simulink model "qless_forgetting_factor_16x16_nofifo"  (R2021a)
settings: Solver=FixedStepDiscrete  StartTime=0.0  StopTime=stoptime*inf  RelTol=1e-3
InitFcn:
  | qless_init_16chan_fi
undefined symbols (not defined in the file): fc, numArrayElements, physconst, srcAngles, Ts
libraries: hdlsllib x137, commfilt2 x4, commrfcorlib x3, commsync2 x3, commrflib2 x2, commrandsrc3 x2, simulink x2, phasedtxrxlib x2, commdigbbndcpm2 x1, embreciprocals x1, commdigbbndpm3 x1
(part 11 of 22)

== system qless_forgetting_factor_16x16_nofifo/MVDR_QLess_HDL/Complex Partial-Systolic Matrix Solve Using Q-less QR Decomposition with Forgetting Factor Manually Tiled n=16/Complex Partial-Systolic Q-less QR with Forgetting Factor/Complex Partial-Systolic Q-less QR with Forgetting Factor Manually tiled/Complex Partial-Systolic Q-less QR Decomposition with Forgetting Factor Section Constant pivot3/Complex Partial-Systolic Q-less QR Row Rotations/Q-less QR Rotate First Element To Real1/Q-less QR Real Row Rotations ==
  x : Inport
  y : Inport  Port=2
  validIn : Inport  Port=3
  restart : Inport  Port=4
  Delay{,1,5..7,10..12,16..18,21} (12 alike) : Delay  DelayLength=1
  Inverse CORDIC Gain : Subsystem  mask(Inverse CORDIC Gain){}
      mask help: fixed:emblib:InverseCORDICGainDescription
      mask Display: disp('1/An')
  Inverse CORDIC Gain1 : Subsystem  mask(Inverse CORDIC Gain){}
      mask help: fixed:emblib:InverseCORDICGainDescription
      mask Display: disp('1/An')
  Q-less QR Real Indexed CORDIC Row Rotation : Subsystem  TreatAsAtomicUnit=on  mask(Real Indexed CORDIC Row Rotation){n=n, pivot=pivot}
      mask prompts: n "fixed:emblib:ColumnsInA"
      mask help: fixed:emblib:RealIdxCORDIC
      mask DialogControl n Prompt: Number of columns in matrix A
  QR 2nd and 3rd Quadrant Compensation : MATLAB Function  TreatAsAtomicUnit=on
  Set Element To Zero : Subsystem  mask(Set Element To Zero){n=n, pivot=pivot}
      mask prompts: n "fixed:emblib:ColumnsInA"
      mask help: fixed:emblib:SetElementToZeroDescription
      mask DialogControl n Prompt: Number of columns in matrix A
  xOut : Outport  VectorParamsAs1DForOutWhenUnconnected=off
  yOut : Outport  Port=2  VectorParamsAs1DForOutWhenUnconnected=off
  validOut : Outport  Port=3  VectorParamsAs1DForOutWhenUnconnected=off
  ready : Outport  Port=4  VectorParamsAs1DForOutWhenUnconnected=off
  wires:
  Delay11/1 -> QR 2nd and 3rd Quadrant Compensation/1(x)
  Delay7/1 -> Set Element To Zero/1(u)
  Delay12/1 -> QR 2nd and 3rd Quadrant Compensation/2(y)
  y/1 -> Delay12/1
  QR 2nd and 3rd Quadrant Compensation/1(xOut) -> Delay/1
  Delay16/1 -> Delay5/1
  Inverse CORDIC Gain1/1(y) -> Delay7/1
  Inverse CORDIC Gain/1(y) -> Delay6/1
  Delay6/1 -> xOut/1
  QR 2nd and 3rd Quadrant Compensation/2(yOut) -> Delay1/1
  x/1 -> Delay11/1
  validIn/1 -> Delay16/1
  Delay17/1 -> Inverse CORDIC Gain/1(u)
  Delay18/1 -> Inverse CORDIC Gain1/1(u)
  Delay21/1 -> Delay10/1
  Set Element To Zero/1(y) -> yOut/1
  Delay10/1 -> validOut/1
  Delay/1 -> Q-less QR Real Indexed CORDIC Row Rotation/1(x)
  Delay1/1 -> Q-less QR Real Indexed CORDIC Row Rotation/2(y)
  Delay5/1 -> Q-less QR Real Indexed CORDIC Row Rotation/3(validIn)
  restart/1 -> Q-less QR Real Indexed CORDIC Row Rotation/4(restart)
  Q-less QR Real Indexed CORDIC Row Rotation/1(xOut) -> Delay17/1
  Q-less QR Real Indexed CORDIC Row Rotation/2(yOut) -> Delay18/1
  Q-less QR Real Indexed CORDIC Row Rotation/3(validOut) -> Delay21/1
  Q-less QR Real Indexed CORDIC Row Rotation/4(ready) -> ready/1

== system qless_forgetting_factor_16x16_nofifo/MVDR_QLess_HDL/Complex Partial-Systolic Matrix Solve Using Q-less QR Decomposition with Forgetting Factor Manually Tiled n=16/Complex Partial-Systolic Q-less QR with Forgetting Factor/Complex Partial-Systolic Q-less QR with Forgetting Factor Manually tiled/Complex Partial-Systolic Q-less QR Decomposition with Forgetting Factor Section Constant pivot3/Complex Partial-Systolic Q-less QR Row Rotations/Q-less QR Rotate First Element To Real1/ValidIn to Ready Logic ==
  readyIn : Inport
  validIn : Inport  Port=2
  AND : Logic  IconShape=distinctive  AllPortsSameDT=off  OutDataTypeStr=boolean
  NOT : Logic  Operator=NOT  IconShape=distinctive  AllPortsSameDT=off  OutDataTypeStr=boolean
  readyOut : Outport  VectorParamsAs1DForOutWhenUnconnected=off
  wires:
  validIn/1 -> NOT/1
  readyIn/1 -> AND/1
  AND/1 -> readyOut/1
  NOT/1 -> AND/2

== system qless_forgetting_factor_16x16_nofifo/MVDR_QLess_HDL/Complex Partial-Systolic Matrix Solve Using Q-less QR Decomposition with Forgetting Factor Manually Tiled n=16/Complex Partial-Systolic Q-less QR with Forgetting Factor/Complex Partial-Systolic Q-less QR with Forgetting Factor Manually tiled/Complex Partial-Systolic Q-less QR Decomposition with Forgetting Factor Section Constant pivot3/Complex Partial-Systolic Q-less QR Row Rotations/Q-less QR Rotate First Element To Real1/ValidIn to Ready Logic1 ==
  readyIn : Inport
  validIn : Inport  Port=2
  AND : Logic  IconShape=distinctive  AllPortsSameDT=off  OutDataTypeStr=boolean
  NOT : Logic  Operator=NOT  IconShape=distinctive  AllPortsSameDT=off  OutDataTypeStr=boolean
  readyOut : Outport  VectorParamsAs1DForOutWhenUnconnected=off
  wires:
  validIn/1 -> NOT/1
  readyIn/1 -> AND/1
  AND/1 -> readyOut/1
  NOT/1 -> AND/2

== system qless_forgetting_factor_16x16_nofifo/MVDR_QLess_HDL/Complex Partial-Systolic Matrix Solve Using Q-less QR Decomposition with Forgetting Factor Manually Tiled n=16/Complex Partial-Systolic Q-less QR with Forgetting Factor/Complex Partial-Systolic Q-less QR with Forgetting Factor Manually tiled/Complex Partial-Systolic Q-less QR Decomposition with Forgetting Factor Section Constant pivot4/Complex Partial-Systolic Q-less QR Row Rotations/Q-less QR Rotate First Element To Real1/Q-less QR Real Row Rotations ==
  x : Inport
  y : Inport  Port=2
  validIn : Inport  Port=3
  restart : Inport  Port=4
  Delay{,1,5..7,10..12,16..18,21} (12 alike) : Delay  DelayLength=1
  Inverse CORDIC Gain : Subsystem  mask(Inverse CORDIC Gain){}
      mask help: fixed:emblib:InverseCORDICGainDescription
      mask Display: disp('1/An')
  Inverse CORDIC Gain1 : Subsystem  mask(Inverse CORDIC Gain){}
      mask help: fixed:emblib:InverseCORDICGainDescription
      mask Display: disp('1/An')
  Q-less QR Real Indexed CORDIC Row Rotation : Subsystem  TreatAsAtomicUnit=on  mask(Real Indexed CORDIC Row Rotation){n=n, pivot=pivot}
      mask prompts: n "fixed:emblib:ColumnsInA"
      mask help: fixed:emblib:RealIdxCORDIC
      mask DialogControl n Prompt: Number of columns in matrix A
  QR 2nd and 3rd Quadrant Compensation : MATLAB Function  TreatAsAtomicUnit=on
  Set Element To Zero : Subsystem  mask(Set Element To Zero){n=n, pivot=pivot}
      mask prompts: n "fixed:emblib:ColumnsInA"
      mask help: fixed:emblib:SetElementToZeroDescription
      mask DialogControl n Prompt: Number of columns in matrix A
  xOut : Outport  VectorParamsAs1DForOutWhenUnconnected=off
  yOut : Outport  Port=2  VectorParamsAs1DForOutWhenUnconnected=off
  validOut : Outport  Port=3  VectorParamsAs1DForOutWhenUnconnected=off
  ready : Outport  Port=4  VectorParamsAs1DForOutWhenUnconnected=off
  wires:
  Delay11/1 -> QR 2nd and 3rd Quadrant Compensation/1(x)
  Delay7/1 -> Set Element To Zero/1(u)
  Delay12/1 -> QR 2nd and 3rd Quadrant Compensation/2(y)
  y/1 -> Delay12/1
  QR 2nd and 3rd Quadrant Compensation/1(xOut) -> Delay/1
  Delay16/1 -> Delay5/1
  Inverse CORDIC Gain1/1(y) -> Delay7/1
  Inverse CORDIC Gain/1(y) -> Delay6/1
  Delay6/1 -> xOut/1
  QR 2nd and 3rd Quadrant Compensation/2(yOut) -> Delay1/1
  x/1 -> Delay11/1
  validIn/1 -> Delay16/1
  Delay17/1 -> Inverse CORDIC Gain/1(u)
  Delay18/1 -> Inverse CORDIC Gain1/1(u)
  Delay21/1 -> Delay10/1
  Set Element To Zero/1(y) -> yOut/1
  Delay10/1 -> validOut/1
  Delay/1 -> Q-less QR Real Indexed CORDIC Row Rotation/1(x)
  Delay1/1 -> Q-less QR Real Indexed CORDIC Row Rotation/2(y)
  Delay5/1 -> Q-less QR Real Indexed CORDIC Row Rotation/3(validIn)
  restart/1 -> Q-less QR Real Indexed CORDIC Row Rotation/4(restart)
  Q-less QR Real Indexed CORDIC Row Rotation/1(xOut) -> Delay17/1
  Q-less QR Real Indexed CORDIC Row Rotation/2(yOut) -> Delay18/1
  Q-less QR Real Indexed CORDIC Row Rotation/3(validOut) -> Delay21/1
  Q-less QR Real Indexed CORDIC Row Rotation/4(ready) -> ready/1

== system qless_forgetting_factor_16x16_nofifo/MVDR_QLess_HDL/Complex Partial-Systolic Matrix Solve Using Q-less QR Decomposition with Forgetting Factor Manually Tiled n=16/Complex Partial-Systolic Q-less QR with Forgetting Factor/Complex Partial-Systolic Q-less QR with Forgetting Factor Manually tiled/Complex Partial-Systolic Q-less QR Decomposition with Forgetting Factor Section Constant pivot4/Complex Partial-Systolic Q-less QR Row Rotations/Q-less QR Rotate First Element To Real1/ValidIn to Ready Logic ==
  readyIn : Inport
  validIn : Inport  Port=2
  AND : Logic  IconShape=distinctive  AllPortsSameDT=off  OutDataTypeStr=boolean
  NOT : Logic  Operator=NOT  IconShape=distinctive  AllPortsSameDT=off  OutDataTypeStr=boolean
  readyOut : Outport  VectorParamsAs1DForOutWhenUnconnected=off
  wires:
  validIn/1 -> NOT/1
  readyIn/1 -> AND/1
  AND/1 -> readyOut/1
  NOT/1 -> AND/2

== system qless_forgetting_factor_16x16_nofifo/MVDR_QLess_HDL/Complex Partial-Systolic Matrix Solve Using Q-less QR Decomposition with Forgetting Factor Manually Tiled n=16/Complex Partial-Systolic Q-less QR with Forgetting Factor/Complex Partial-Systolic Q-less QR with Forgetting Factor Manually tiled/Complex Partial-Systolic Q-less QR Decomposition with Forgetting Factor Section Constant pivot4/Complex Partial-Systolic Q-less QR Row Rotations/Q-less QR Rotate First Element To Real1/ValidIn to Ready Logic1 ==
  readyIn : Inport
  validIn : Inport  Port=2
  AND : Logic  IconShape=distinctive  AllPortsSameDT=off  OutDataTypeStr=boolean
  NOT : Logic  Operator=NOT  IconShape=distinctive  AllPortsSameDT=off  OutDataTypeStr=boolean
  readyOut : Outport  VectorParamsAs1DForOutWhenUnconnected=off
  wires:
  validIn/1 -> NOT/1
  readyIn/1 -> AND/1
  AND/1 -> readyOut/1
  NOT/1 -> AND/2

== system qless_forgetting_factor_16x16_nofifo/MVDR_QLess_HDL/Complex Partial-Systolic Matrix Solve Using Q-less QR Decomposition with Forgetting Factor Manually Tiled n=16/Complex Partial-Systolic Q-less QR with Forgetting Factor/Complex Partial-Systolic Q-less QR with Forgetting Factor Manually tiled/Complex Partial-Systolic Q-less QR Decomposition with Forgetting Factor Section Constant pivot5/Complex Partial-Systolic Q-less QR Row Rotations/Q-less QR Rotate First Element To Real1/Q-less QR Real Row Rotations ==
  x : Inport
  y : Inport  Port=2
  validIn : Inport  Port=3
  restart : Inport  Port=4
  Delay{,1,5..7,10..12,16..18,21} (12 alike) : Delay  DelayLength=1
  Inverse CORDIC Gain : Subsystem  mask(Inverse CORDIC Gain){}
      mask help: fixed:emblib:InverseCORDICGainDescription
      mask Display: disp('1/An')
  Inverse CORDIC Gain1 : Subsystem  mask(Inverse CORDIC Gain){}
      mask help: fixed:emblib:InverseCORDICGainDescription
      mask Display: disp('1/An')
  Q-less QR Real Indexed CORDIC Row Rotation : Subsystem  TreatAsAtomicUnit=on  mask(Real Indexed CORDIC Row Rotation){n=n, pivot=pivot}
      mask prompts: n "fixed:emblib:ColumnsInA"
      mask help: fixed:emblib:RealIdxCORDIC
      mask DialogControl n Prompt: Number of columns in matrix A
  QR 2nd and 3rd Quadrant Compensation : MATLAB Function  TreatAsAtomicUnit=on
  Set Element To Zero : Subsystem  mask(Set Element To Zero){n=n, pivot=pivot}
      mask prompts: n "fixed:emblib:ColumnsInA"
      mask help: fixed:emblib:SetElementToZeroDescription
      mask DialogControl n Prompt: Number of columns in matrix A
  xOut : Outport  VectorParamsAs1DForOutWhenUnconnected=off
  yOut : Outport  Port=2  VectorParamsAs1DForOutWhenUnconnected=off
  validOut : Outport  Port=3  VectorParamsAs1DForOutWhenUnconnected=off
  ready : Outport  Port=4  VectorParamsAs1DForOutWhenUnconnected=off
  wires:
  Delay11/1 -> QR 2nd and 3rd Quadrant Compensation/1(x)
  Delay7/1 -> Set Element To Zero/1(u)
  Delay12/1 -> QR 2nd and 3rd Quadrant Compensation/2(y)
  y/1 -> Delay12/1
  QR 2nd and 3rd Quadrant Compensation/1(xOut) -> Delay/1
  Delay16/1 -> Delay5/1
  Inverse CORDIC Gain1/1(y) -> Delay7/1
  Inverse CORDIC Gain/1(y) -> Delay6/1
  Delay6/1 -> xOut/1
  QR 2nd and 3rd Quadrant Compensation/2(yOut) -> Delay1/1
  x/1 -> Delay11/1
  validIn/1 -> Delay16/1
  Delay17/1 -> Inverse CORDIC Gain/1(u)
  Delay18/1 -> Inverse CORDIC Gain1/1(u)
  Delay21/1 -> Delay10/1
  Set Element To Zero/1(y) -> yOut/1
  Delay10/1 -> validOut/1
  Delay/1 -> Q-less QR Real Indexed CORDIC Row Rotation/1(x)
  Delay1/1 -> Q-less QR Real Indexed CORDIC Row Rotation/2(y)
  Delay5/1 -> Q-less QR Real Indexed CORDIC Row Rotation/3(validIn)
  restart/1 -> Q-less QR Real Indexed CORDIC Row Rotation/4(restart)
  Q-less QR Real Indexed CORDIC Row Rotation/1(xOut) -> Delay17/1
  Q-less QR Real Indexed CORDIC Row Rotation/2(yOut) -> Delay18/1
  Q-less QR Real Indexed CORDIC Row Rotation/3(validOut) -> Delay21/1
  Q-less QR Real Indexed CORDIC Row Rotation/4(ready) -> ready/1

== system qless_forgetting_factor_16x16_nofifo/MVDR_QLess_HDL/Complex Partial-Systolic Matrix Solve Using Q-less QR Decomposition with Forgetting Factor Manually Tiled n=16/Complex Partial-Systolic Q-less QR with Forgetting Factor/Complex Partial-Systolic Q-less QR with Forgetting Factor Manually tiled/Complex Partial-Systolic Q-less QR Decomposition with Forgetting Factor Section Constant pivot5/Complex Partial-Systolic Q-less QR Row Rotations/Q-less QR Rotate First Element To Real1/ValidIn to Ready Logic ==
  readyIn : Inport
  validIn : Inport  Port=2
  AND : Logic  IconShape=distinctive  AllPortsSameDT=off  OutDataTypeStr=boolean
  NOT : Logic  Operator=NOT  IconShape=distinctive  AllPortsSameDT=off  OutDataTypeStr=boolean
  readyOut : Outport  VectorParamsAs1DForOutWhenUnconnected=off
  wires:
  validIn/1 -> NOT/1
  readyIn/1 -> AND/1
  AND/1 -> readyOut/1
  NOT/1 -> AND/2

== system qless_forgetting_factor_16x16_nofifo/MVDR_QLess_HDL/Complex Partial-Systolic Matrix Solve Using Q-less QR Decomposition with Forgetting Factor Manually Tiled n=16/Complex Partial-Systolic Q-less QR with Forgetting Factor/Complex Partial-Systolic Q-less QR with Forgetting Factor Manually tiled/Complex Partial-Systolic Q-less QR Decomposition with Forgetting Factor Section Constant pivot5/Complex Partial-Systolic Q-less QR Row Rotations/Q-less QR Rotate First Element To Real1/ValidIn to Ready Logic1 ==
  readyIn : Inport
  validIn : Inport  Port=2
  AND : Logic  IconShape=distinctive  AllPortsSameDT=off  OutDataTypeStr=boolean
  NOT : Logic  Operator=NOT  IconShape=distinctive  AllPortsSameDT=off  OutDataTypeStr=boolean
  readyOut : Outport  VectorParamsAs1DForOutWhenUnconnected=off
  wires:
  validIn/1 -> NOT/1
  readyIn/1 -> AND/1
  AND/1 -> readyOut/1
  NOT/1 -> AND/2

== system qless_forgetting_factor_16x16_nofifo/MVDR_QLess_HDL/Complex Partial-Systolic Matrix Solve Using Q-less QR Decomposition with Forgetting Factor Manually Tiled n=16/Complex Partial-Systolic Q-less QR with Forgetting Factor/Complex Partial-Systolic Q-less QR with Forgetting Factor Manually tiled/Complex Partial-Systolic Q-less QR Decomposition with Forgetting Factor Section Constant pivot6/Complex Partial-Systolic Q-less QR Row Rotations/Q-less QR Rotate First Element To Real1/Q-less QR Real Row Rotations ==
  x : Inport
  y : Inport  Port=2
  validIn : Inport  Port=3
  restart : Inport  Port=4
  Delay{,1,5..7,10..12,16..18,21} (12 alike) : Delay  DelayLength=1
  Inverse CORDIC Gain : Subsystem  mask(Inverse CORDIC Gain){}
      mask help: fixed:emblib:InverseCORDICGainDescription
      mask Display: disp('1/An')
  Inverse CORDIC Gain1 : Subsystem  mask(Inverse CORDIC Gain){}
      mask help: fixed:emblib:InverseCORDICGainDescription
      mask Display: disp('1/An')
  Q-less QR Real Indexed CORDIC Row Rotation : Subsystem  TreatAsAtomicUnit=on  mask(Real Indexed CORDIC Row Rotation){n=n, pivot=pivot}
      mask prompts: n "fixed:emblib:ColumnsInA"
      mask help: fixed:emblib:RealIdxCORDIC
      mask DialogControl n Prompt: Number of columns in matrix A
  QR 2nd and 3rd Quadrant Compensation : MATLAB Function  TreatAsAtomicUnit=on
  Set Element To Zero : Subsystem  mask(Set Element To Zero){n=n, pivot=pivot}
      mask prompts: n "fixed:emblib:ColumnsInA"
      mask help: fixed:emblib:SetElementToZeroDescription
      mask DialogControl n Prompt: Number of columns in matrix A
  xOut : Outport  VectorParamsAs1DForOutWhenUnconnected=off
  yOut : Outport  Port=2  VectorParamsAs1DForOutWhenUnconnected=off
  validOut : Outport  Port=3  VectorParamsAs1DForOutWhenUnconnected=off
  ready : Outport  Port=4  VectorParamsAs1DForOutWhenUnconnected=off
  wires:
  Delay11/1 -> QR 2nd and 3rd Quadrant Compensation/1(x)
  Delay7/1 -> Set Element To Zero/1(u)
  Delay12/1 -> QR 2nd and 3rd Quadrant Compensation/2(y)
  y/1 -> Delay12/1
  QR 2nd and 3rd Quadrant Compensation/1(xOut) -> Delay/1
  Delay16/1 -> Delay5/1
  Inverse CORDIC Gain1/1(y) -> Delay7/1
  Inverse CORDIC Gain/1(y) -> Delay6/1
  Delay6/1 -> xOut/1
  QR 2nd and 3rd Quadrant Compensation/2(yOut) -> Delay1/1
  x/1 -> Delay11/1
  validIn/1 -> Delay16/1
  Delay17/1 -> Inverse CORDIC Gain/1(u)
  Delay18/1 -> Inverse CORDIC Gain1/1(u)
  Delay21/1 -> Delay10/1
  Set Element To Zero/1(y) -> yOut/1
  Delay10/1 -> validOut/1
  Delay/1 -> Q-less QR Real Indexed CORDIC Row Rotation/1(x)
  Delay1/1 -> Q-less QR Real Indexed CORDIC Row Rotation/2(y)
  Delay5/1 -> Q-less QR Real Indexed CORDIC Row Rotation/3(validIn)
  restart/1 -> Q-less QR Real Indexed CORDIC Row Rotation/4(restart)
  Q-less QR Real Indexed CORDIC Row Rotation/1(xOut) -> Delay17/1
  Q-less QR Real Indexed CORDIC Row Rotation/2(yOut) -> Delay18/1
  Q-less QR Real Indexed CORDIC Row Rotation/3(validOut) -> Delay21/1
  Q-less QR Real Indexed CORDIC Row Rotation/4(ready) -> ready/1

== system qless_forgetting_factor_16x16_nofifo/MVDR_QLess_HDL/Complex Partial-Systolic Matrix Solve Using Q-less QR Decomposition with Forgetting Factor Manually Tiled n=16/Complex Partial-Systolic Q-less QR with Forgetting Factor/Complex Partial-Systolic Q-less QR with Forgetting Factor Manually tiled/Complex Partial-Systolic Q-less QR Decomposition with Forgetting Factor Section Constant pivot6/Complex Partial-Systolic Q-less QR Row Rotations/Q-less QR Rotate First Element To Real1/ValidIn to Ready Logic ==
  readyIn : Inport
  validIn : Inport  Port=2
  AND : Logic  IconShape=distinctive  AllPortsSameDT=off  OutDataTypeStr=boolean
  NOT : Logic  Operator=NOT  IconShape=distinctive  AllPortsSameDT=off  OutDataTypeStr=boolean
  readyOut : Outport  VectorParamsAs1DForOutWhenUnconnected=off
  wires:
  validIn/1 -> NOT/1
  readyIn/1 -> AND/1
  AND/1 -> readyOut/1
  NOT/1 -> AND/2

== system qless_forgetting_factor_16x16_nofifo/MVDR_QLess_HDL/Complex Partial-Systolic Matrix Solve Using Q-less QR Decomposition with Forgetting Factor Manually Tiled n=16/Complex Partial-Systolic Q-less QR with Forgetting Factor/Complex Partial-Systolic Q-less QR with Forgetting Factor Manually tiled/Complex Partial-Systolic Q-less QR Decomposition with Forgetting Factor Section Constant pivot6/Complex Partial-Systolic Q-less QR Row Rotations/Q-less QR Rotate First Element To Real1/ValidIn to Ready Logic1 ==
  readyIn : Inport
  validIn : Inport  Port=2
  AND : Logic  IconShape=distinctive  AllPortsSameDT=off  OutDataTypeStr=boolean
  NOT : Logic  Operator=NOT  IconShape=distinctive  AllPortsSameDT=off  OutDataTypeStr=boolean
  readyOut : Outport  VectorParamsAs1DForOutWhenUnconnected=off
  wires:
  validIn/1 -> NOT/1
  readyIn/1 -> AND/1
  AND/1 -> readyOut/1
  NOT/1 -> AND/2

== system qless_forgetting_factor_16x16_nofifo/MVDR_QLess_HDL/Complex Partial-Systolic Matrix Solve Using Q-less QR Decomposition with Forgetting Factor Manually Tiled n=16/Complex Partial-Systolic Q-less QR with Forgetting Factor/Complex Partial-Systolic Q-less QR with Forgetting Factor Manually tiled/Complex Partial-Systolic Q-less QR Decomposition with Forgetting Factor Section Constant pivot7/Complex Partial-Systolic Q-less QR Row Rotations/Q-less QR Rotate First Element To Real1/Q-less QR Real Row Rotations ==
  x : Inport
  y : Inport  Port=2
  validIn : Inport  Port=3
  restart : Inport  Port=4
  Delay{,1,5..7,10..12,16..18,21} (12 alike) : Delay  DelayLength=1
  Inverse CORDIC Gain : Subsystem  mask(Inverse CORDIC Gain){}
      mask help: fixed:emblib:InverseCORDICGainDescription
      mask Display: disp('1/An')
  Inverse CORDIC Gain1 : Subsystem  mask(Inverse CORDIC Gain){}
      mask help: fixed:emblib:InverseCORDICGainDescription
      mask Display: disp('1/An')
  Q-less QR Real Indexed CORDIC Row Rotation : Subsystem  TreatAsAtomicUnit=on  mask(Real Indexed CORDIC Row Rotation){n=n, pivot=pivot}
      mask prompts: n "fixed:emblib:ColumnsInA"
      mask help: fixed:emblib:RealIdxCORDIC
      mask DialogControl n Prompt: Number of columns in matrix A
  QR 2nd and 3rd Quadrant Compensation : MATLAB Function  TreatAsAtomicUnit=on
  Set Element To Zero : Subsystem  mask(Set Element To Zero){n=n, pivot=pivot}
      mask prompts: n "fixed:emblib:ColumnsInA"
      mask help: fixed:emblib:SetElementToZeroDescription
      mask DialogControl n Prompt: Number of columns in matrix A
  xOut : Outport  VectorParamsAs1DForOutWhenUnconnected=off
  yOut : Outport  Port=2  VectorParamsAs1DForOutWhenUnconnected=off
  validOut : Outport  Port=3  VectorParamsAs1DForOutWhenUnconnected=off
  ready : Outport  Port=4  VectorParamsAs1DForOutWhenUnconnected=off
  wires:
  Delay11/1 -> QR 2nd and 3rd Quadrant Compensation/1(x)
  Delay7/1 -> Set Element To Zero/1(u)
  Delay12/1 -> QR 2nd and 3rd Quadrant Compensation/2(y)
  y/1 -> Delay12/1
  QR 2nd and 3rd Quadrant Compensation/1(xOut) -> Delay/1
  Delay16/1 -> Delay5/1
  Inverse CORDIC Gain1/1(y) -> Delay7/1
  Inverse CORDIC Gain/1(y) -> Delay6/1
  Delay6/1 -> xOut/1
  QR 2nd and 3rd Quadrant Compensation/2(yOut) -> Delay1/1
  x/1 -> Delay11/1
  validIn/1 -> Delay16/1
  Delay17/1 -> Inverse CORDIC Gain/1(u)
  Delay18/1 -> Inverse CORDIC Gain1/1(u)
  Delay21/1 -> Delay10/1
  Set Element To Zero/1(y) -> yOut/1
  Delay10/1 -> validOut/1
  Delay/1 -> Q-less QR Real Indexed CORDIC Row Rotation/1(x)
  Delay1/1 -> Q-less QR Real Indexed CORDIC Row Rotation/2(y)
  Delay5/1 -> Q-less QR Real Indexed CORDIC Row Rotation/3(validIn)
  restart/1 -> Q-less QR Real Indexed CORDIC Row Rotation/4(restart)
  Q-less QR Real Indexed CORDIC Row Rotation/1(xOut) -> Delay17/1
  Q-less QR Real Indexed CORDIC Row Rotation/2(yOut) -> Delay18/1
  Q-less QR Real Indexed CORDIC Row Rotation/3(validOut) -> Delay21/1
  Q-less QR Real Indexed CORDIC Row Rotation/4(ready) -> ready/1

== system qless_forgetting_factor_16x16_nofifo/MVDR_QLess_HDL/Complex Partial-Systolic Matrix Solve Using Q-less QR Decomposition with Forgetting Factor Manually Tiled n=16/Complex Partial-Systolic Q-less QR with Forgetting Factor/Complex Partial-Systolic Q-less QR with Forgetting Factor Manually tiled/Complex Partial-Systolic Q-less QR Decomposition with Forgetting Factor Section Constant pivot7/Complex Partial-Systolic Q-less QR Row Rotations/Q-less QR Rotate First Element To Real1/ValidIn to Ready Logic ==
  readyIn : Inport
  validIn : Inport  Port=2
  AND : Logic  IconShape=distinctive  AllPortsSameDT=off  OutDataTypeStr=boolean
  NOT : Logic  Operator=NOT  IconShape=distinctive  AllPortsSameDT=off  OutDataTypeStr=boolean
  readyOut : Outport  VectorParamsAs1DForOutWhenUnconnected=off
  wires:
  validIn/1 -> NOT/1
  readyIn/1 -> AND/1
  AND/1 -> readyOut/1
  NOT/1 -> AND/2

== system qless_forgetting_factor_16x16_nofifo/MVDR_QLess_HDL/Complex Partial-Systolic Matrix Solve Using Q-less QR Decomposition with Forgetting Factor Manually Tiled n=16/Complex Partial-Systolic Q-less QR with Forgetting Factor/Complex Partial-Systolic Q-less QR with Forgetting Factor Manually tiled/Complex Partial-Systolic Q-less QR Decomposition with Forgetting Factor Section Constant pivot7/Complex Partial-Systolic Q-less QR Row Rotations/Q-less QR Rotate First Element To Real1/ValidIn to Ready Logic1 ==
  readyIn : Inport
  validIn : Inport  Port=2
  AND : Logic  IconShape=distinctive  AllPortsSameDT=off  OutDataTypeStr=boolean
  NOT : Logic  Operator=NOT  IconShape=distinctive  AllPortsSameDT=off  OutDataTypeStr=boolean
  readyOut : Outport  VectorParamsAs1DForOutWhenUnconnected=off
  wires:
  validIn/1 -> NOT/1
  readyIn/1 -> AND/1
  AND/1 -> readyOut/1
  NOT/1 -> AND/2

== system qless_forgetting_factor_16x16_nofifo/MVDR_QLess_HDL/Complex Partial-Systolic Matrix Solve Using Q-less QR Decomposition with Forgetting Factor Manually Tiled n=16/Complex Partial-Systolic Q-less QR with Forgetting Factor/Complex Partial-Systolic Q-less QR with Forgetting Factor Manually tiled/Complex Partial-Systolic Q-less QR Decomposition with Forgetting Factor Section Constant pivot8/Complex Partial-Systolic Q-less QR Row Rotations/Q-less QR Rotate First Element To Real1/Q-less QR Real Row Rotations ==
  x : Inport
  y : Inport  Port=2
  validIn : Inport  Port=3
  restart : Inport  Port=4
  Delay{,1,5..7,10..12,16..18,21} (12 alike) : Delay  DelayLength=1
  Inverse CORDIC Gain : Subsystem  mask(Inverse CORDIC Gain){}
      mask help: fixed:emblib:InverseCORDICGainDescription
      mask Display: disp('1/An')
  Inverse CORDIC Gain1 : Subsystem  mask(Inverse CORDIC Gain){}
      mask help: fixed:emblib:InverseCORDICGainDescription
      mask Display: disp('1/An')
  Q-less QR Real Indexed CORDIC Row Rotation : Subsystem  TreatAsAtomicUnit=on  mask(Real Indexed CORDIC Row Rotation){n=n, pivot=pivot}
      mask prompts: n "fixed:emblib:ColumnsInA"
      mask help: fixed:emblib:RealIdxCORDIC
      mask DialogControl n Prompt: Number of columns in matrix A
  QR 2nd and 3rd Quadrant Compensation : MATLAB Function  TreatAsAtomicUnit=on
  Set Element To Zero : Subsystem  mask(Set Element To Zero){n=n, pivot=pivot}
      mask prompts: n "fixed:emblib:ColumnsInA"
      mask help: fixed:emblib:SetElementToZeroDescription
      mask DialogControl n Prompt: Number of columns in matrix A
  xOut : Outport  VectorParamsAs1DForOutWhenUnconnected=off
  yOut : Outport  Port=2  VectorParamsAs1DForOutWhenUnconnected=off
  validOut : Outport  Port=3  VectorParamsAs1DForOutWhenUnconnected=off
  ready : Outport  Port=4  VectorParamsAs1DForOutWhenUnconnected=off
  wires:
  Delay11/1 -> QR 2nd and 3rd Quadrant Compensation/1(x)
  Delay7/1 -> Set Element To Zero/1(u)
  Delay12/1 -> QR 2nd and 3rd Quadrant Compensation/2(y)
  y/1 -> Delay12/1
  QR 2nd and 3rd Quadrant Compensation/1(xOut) -> Delay/1
  Delay16/1 -> Delay5/1
  Inverse CORDIC Gain1/1(y) -> Delay7/1
  Inverse CORDIC Gain/1(y) -> Delay6/1
  Delay6/1 -> xOut/1
  QR 2nd and 3rd Quadrant Compensation/2(yOut) -> Delay1/1
  x/1 -> Delay11/1
  validIn/1 -> Delay16/1
  Delay17/1 -> Inverse CORDIC Gain/1(u)
  Delay18/1 -> Inverse CORDIC Gain1/1(u)
  Delay21/1 -> Delay10/1
  Set Element To Zero/1(y) -> yOut/1
  Delay10/1 -> validOut/1
  Delay/1 -> Q-less QR Real Indexed CORDIC Row Rotation/1(x)
  Delay1/1 -> Q-less QR Real Indexed CORDIC Row Rotation/2(y)
  Delay5/1 -> Q-less QR Real Indexed CORDIC Row Rotation/3(validIn)
  restart/1 -> Q-less QR Real Indexed CORDIC Row Rotation/4(restart)
  Q-less QR Real Indexed CORDIC Row Rotation/1(xOut) -> Delay17/1
  Q-less QR Real Indexed CORDIC Row Rotation/2(yOut) -> Delay18/1
  Q-less QR Real Indexed CORDIC Row Rotation/3(validOut) -> Delay21/1
  Q-less QR Real Indexed CORDIC Row Rotation/4(ready) -> ready/1

== system qless_forgetting_factor_16x16_nofifo/MVDR_QLess_HDL/Complex Partial-Systolic Matrix Solve Using Q-less QR Decomposition with Forgetting Factor Manually Tiled n=16/Complex Partial-Systolic Q-less QR with Forgetting Factor/Complex Partial-Systolic Q-less QR with Forgetting Factor Manually tiled/Complex Partial-Systolic Q-less QR Decomposition with Forgetting Factor Section Constant pivot8/Complex Partial-Systolic Q-less QR Row Rotations/Q-less QR Rotate First Element To Real1/ValidIn to Ready Logic ==
  readyIn : Inport
  validIn : Inport  Port=2
  AND : Logic  IconShape=distinctive  AllPortsSameDT=off  OutDataTypeStr=boolean
  NOT : Logic  Operator=NOT  IconShape=distinctive  AllPortsSameDT=off  OutDataTypeStr=boolean
  readyOut : Outport  VectorParamsAs1DForOutWhenUnconnected=off
  wires:
  validIn/1 -> NOT/1
  readyIn/1 -> AND/1
  AND/1 -> readyOut/1
  NOT/1 -> AND/2

== system qless_forgetting_factor_16x16_nofifo/MVDR_QLess_HDL/Complex Partial-Systolic Matrix Solve Using Q-less QR Decomposition with Forgetting Factor Manually Tiled n=16/Complex Partial-Systolic Q-less QR with Forgetting Factor/Complex Partial-Systolic Q-less QR with Forgetting Factor Manually tiled/Complex Partial-Systolic Q-less QR Decomposition with Forgetting Factor Section Constant pivot8/Complex Partial-Systolic Q-less QR Row Rotations/Q-less QR Rotate First Element To Real1/ValidIn to Ready Logic1 ==
  readyIn : Inport
  validIn : Inport  Port=2
  AND : Logic  IconShape=distinctive  AllPortsSameDT=off  OutDataTypeStr=boolean
  NOT : Logic  Operator=NOT  IconShape=distinctive  AllPortsSameDT=off  OutDataTypeStr=boolean
  readyOut : Outport  VectorParamsAs1DForOutWhenUnconnected=off
  wires:
  validIn/1 -> NOT/1
  readyIn/1 -> AND/1
  AND/1 -> readyOut/1
  NOT/1 -> AND/2

== system qless_forgetting_factor_16x16_nofifo/MVDR_QLess_HDL/Complex Partial-Systolic Matrix Solve Using Q-less QR Decomposition with Forgetting Factor Manually Tiled n=16/Complex Partial-Systolic Q-less QR with Forgetting Factor/Complex Partial-Systolic Q-less QR with Forgetting Factor Manually tiled/Complex Partial-Systolic Q-less QR Decomposition with Forgetting Factor Section Constant pivot9/Complex Partial-Systolic Q-less QR Row Rotations/Q-less QR Rotate First Element To Real1/Q-less QR Real Row Rotations ==
  x : Inport
  y : Inport  Port=2
  validIn : Inport  Port=3
  restart : Inport  Port=4
  Delay{,1,5..7,10..12,16..18,21} (12 alike) : Delay  DelayLength=1
  Inverse CORDIC Gain : Subsystem  mask(Inverse CORDIC Gain){}
      mask help: fixed:emblib:InverseCORDICGainDescription
      mask Display: disp('1/An')
  Inverse CORDIC Gain1 : Subsystem  mask(Inverse CORDIC Gain){}
      mask help: fixed:emblib:InverseCORDICGainDescription
      mask Display: disp('1/An')
  Q-less QR Real Indexed CORDIC Row Rotation : Subsystem  TreatAsAtomicUnit=on  mask(Real Indexed CORDIC Row Rotation){n=n, pivot=pivot}
      mask prompts: n "fixed:emblib:ColumnsInA"
      mask help: fixed:emblib:RealIdxCORDIC
      mask DialogControl n Prompt: Number of columns in matrix A
  QR 2nd and 3rd Quadrant Compensation : MATLAB Function  TreatAsAtomicUnit=on
  Set Element To Zero : Subsystem  mask(Set Element To Zero){n=n, pivot=pivot}
      mask prompts: n "fixed:emblib:ColumnsInA"
      mask help: fixed:emblib:SetElementToZeroDescription
      mask DialogControl n Prompt: Number of columns in matrix A
  xOut : Outport  VectorParamsAs1DForOutWhenUnconnected=off
  yOut : Outport  Port=2  VectorParamsAs1DForOutWhenUnconnected=off
  validOut : Outport  Port=3  VectorParamsAs1DForOutWhenUnconnected=off
  ready : Outport  Port=4  VectorParamsAs1DForOutWhenUnconnected=off
  wires:
  Delay11/1 -> QR 2nd and 3rd Quadrant Compensation/1(x)
  Delay7/1 -> Set Element To Zero/1(u)
  Delay12/1 -> QR 2nd and 3rd Quadrant Compensation/2(y)
  y/1 -> Delay12/1
  QR 2nd and 3rd Quadrant Compensation/1(xOut) -> Delay/1
  Delay16/1 -> Delay5/1
  Inverse CORDIC Gain1/1(y) -> Delay7/1
  Inverse CORDIC Gain/1(y) -> Delay6/1
  Delay6/1 -> xOut/1
  QR 2nd and 3rd Quadrant Compensation/2(yOut) -> Delay1/1
  x/1 -> Delay11/1
  validIn/1 -> Delay16/1
  Delay17/1 -> Inverse CORDIC Gain/1(u)
  Delay18/1 -> Inverse CORDIC Gain1/1(u)
  Delay21/1 -> Delay10/1
  Set Element To Zero/1(y) -> yOut/1
  Delay10/1 -> validOut/1
  Delay/1 -> Q-less QR Real Indexed CORDIC Row Rotation/1(x)
  Delay1/1 -> Q-less QR Real Indexed CORDIC Row Rotation/2(y)
  Delay5/1 -> Q-less QR Real Indexed CORDIC Row Rotation/3(validIn)
  restart/1 -> Q-less QR Real Indexed CORDIC Row Rotation/4(restart)
  Q-less QR Real Indexed CORDIC Row Rotation/1(xOut) -> Delay17/1
  Q-less QR Real Indexed CORDIC Row Rotation/2(yOut) -> Delay18/1
  Q-less QR Real Indexed CORDIC Row Rotation/3(validOut) -> Delay21/1
  Q-less QR Real Indexed CORDIC Row Rotation/4(ready) -> ready/1

== system qless_forgetting_factor_16x16_nofifo/MVDR_QLess_HDL/Complex Partial-Systolic Matrix Solve Using Q-less QR Decomposition with Forgetting Factor Manually Tiled n=16/Complex Partial-Systolic Q-less QR with Forgetting Factor/Complex Partial-Systolic Q-less QR with Forgetting Factor Manually tiled/Complex Partial-Systolic Q-less QR Decomposition with Forgetting Factor Section Constant pivot9/Complex Partial-Systolic Q-less QR Row Rotations/Q-less QR Rotate First Element To Real1/ValidIn to Ready Logic ==
  readyIn : Inport
  validIn : Inport  Port=2
  AND : Logic  IconShape=distinctive  AllPortsSameDT=off  OutDataTypeStr=boolean
  NOT : Logic  Operator=NOT  IconShape=distinctive  AllPortsSameDT=off  OutDataTypeStr=boolean
  readyOut : Outport  VectorParamsAs1DForOutWhenUnconnected=off
  wires:
  validIn/1 -> NOT/1
  readyIn/1 -> AND/1
  AND/1 -> readyOut/1
  NOT/1 -> AND/2

== system qless_forgetting_factor_16x16_nofifo/MVDR_QLess_HDL/Complex Partial-Systolic Matrix Solve Using Q-less QR Decomposition with Forgetting Factor Manually Tiled n=16/Complex Partial-Systolic Q-less QR with Forgetting Factor/Complex Partial-Systolic Q-less QR with Forgetting Factor Manually tiled/Complex Partial-Systolic Q-less QR Decomposition with Forgetting Factor Section Constant pivot9/Complex Partial-Systolic Q-less QR Row Rotations/Q-less QR Rotate First Element To Real1/ValidIn to Ready Logic1 ==
  readyIn : Inport
  validIn : Inport  Port=2
  AND : Logic  IconShape=distinctive  AllPortsSameDT=off  OutDataTypeStr=boolean
  NOT : Logic  Operator=NOT  IconShape=distinctive  AllPortsSameDT=off  OutDataTypeStr=boolean
  readyOut : Outport  VectorParamsAs1DForOutWhenUnconnected=off
  wires:
  validIn/1 -> NOT/1
  readyIn/1 -> AND/1
  AND/1 -> readyOut/1
  NOT/1 -> AND/2

== system qless_forgetting_factor_16x16_nofifo/MVDR_QLess_HDL/Complex Partial-Systolic Matrix Solve Using Q-less QR Decomposition with Forgetting Factor Manually Tiled n=16/Complex Partial-Systolic Q-less QR with Forgetting Factor/Complex Partial-Systolic Q-less QR with Forgetting Factor Manually tiled/Complex Partial-Systolic Q-less QR Decomposition with Forgetting Factor Section Constant pivot1/Complex Partial-Systolic Q-less QR Row Rotations/Q-less QR Rotate First Element To Real1/Q-less QR Real Row Rotations/Inverse CORDIC Gain ==
  u : Inport
  MATLAB Function : MATLAB Function  TreatAsAtomicUnit=on
  y : Outport  VectorParamsAs1DForOutWhenUnconnected=off
  wires:
  MATLAB Function/1(y) -> y/1
  u/1 -> MATLAB Function/1(u)

== system qless_forgetting_factor_16x16_nofifo/MVDR_QLess_HDL/Complex Partial-Systolic Matrix Solve Using Q-less QR Decomposition with Forgetting Factor Manually Tiled n=16/Complex Partial-Systolic Q-less QR with Forgetting Factor/Complex Partial-Systolic Q-less QR with Forgetting Factor Manually tiled/Complex Partial-Systolic Q-less QR Decomposition with Forgetting Factor Section Constant pivot1/Complex Partial-Systolic Q-less QR Row Rotations/Q-less QR Rotate First Element To Real1/Q-less QR Real Row Rotations/Inverse CORDIC Gain1 ==
  u : Inport
  MATLAB Function : MATLAB Function  TreatAsAtomicUnit=on
  y : Outport  VectorParamsAs1DForOutWhenUnconnected=off
  wires:
  MATLAB Function/1(y) -> y/1
  u/1 -> MATLAB Function/1(u)

== system qless_forgetting_factor_16x16_nofifo/MVDR_QLess_HDL/Complex Partial-Systolic Matrix Solve Using Q-less QR Decomposition with Forgetting Factor Manually Tiled n=16/Complex Partial-Systolic Q-less QR with Forgetting Factor/Complex Partial-Systolic Q-less QR with Forgetting Factor Manually tiled/Complex Partial-Systolic Q-less QR Decomposition with Forgetting Factor Section Constant pivot1/Complex Partial-Systolic Q-less QR Row Rotations/Q-less QR Rotate First Element To Real1/Q-less QR Real Row Rotations/Q-less QR Real Indexed CORDIC Row Rotation ==
  x : Inport
  y : Inport  Port=2
  validIn : Inport  Port=3
  restart : Inport  Port=4
  CORDIC QR Kernel : MATLAB Function  TreatAsAtomicUnit=on
  Delay{1..3,6} (4 alike) : Delay  DelayLength=1
  State Control : StateControl  StateControl=Synchronous
  Unit Delay Enabled Synchronous1 : hdlsllib/Discrete/Unit Delay Enabled Synchronous  InitialCondition=0.0  SampleTime=-1
      settings: SourceProductBaseCode=SL
  Unit Delay Enabled Synchronous4 : hdlsllib/Discrete/Unit Delay Enabled Synchronous  InitialCondition=0.0  SampleTime=-1
      settings: SourceProductBaseCode=SL
  xOut : Outport  VectorParamsAs1DForOutWhenUnconnected=off
  yOut : Outport  Port=2  VectorParamsAs1DForOutWhenUnconnected=off
  validOut : Outport  Port=3  VectorParamsAs1DForOutWhenUnconnected=off
  ready : Outport  Port=4  VectorParamsAs1DForOutWhenUnconnected=off
  wires:
  Delay6/1 -> CORDIC QR Kernel/3(validIn)
  Delay2/1 -> CORDIC QR Kernel/2(yIn)
  Delay1/1 -> CORDIC QR Kernel/1(xIn)
  CORDIC QR Kernel/4(ready) -> ready/1
  CORDIC QR Kernel/3(validOut) -> Unit Delay Enabled Synchronous1/2, Unit Delay Enabled Synchronous4/2, Delay3/1
  restart/1 -> CORDIC QR Kernel/4(restart)
  Unit Delay Enabled Synchronous4/1 -> xOut/1
  validIn/1 -> Delay6/1
  CORDIC QR Kernel/2(yOut) -> Unit Delay Enabled Synchronous1/1
  x/1 -> Delay1/1
  y/1 -> Delay2/1
  CORDIC QR Kernel/1(xOut) -> Unit Delay Enabled Synchronous4/1
  Unit Delay Enabled Synchronous1/1 -> yOut/1
  Delay3/1 -> validOut/1

== system qless_forgetting_factor_16x16_nofifo/MVDR_QLess_HDL/Complex Partial-Systolic Matrix Solve Using Q-less QR Decomposition with Forgetting Factor Manually Tiled n=16/Complex Partial-Systolic Q-less QR with Forgetting Factor/Complex Partial-Systolic Q-less QR with Forgetting Factor Manually tiled/Complex Partial-Systolic Q-less QR Decomposition with Forgetting Factor Section Constant pivot1/Complex Partial-Systolic Q-less QR Row Rotations/Q-less QR Rotate First Element To Real1/Q-less QR Real Row Rotations/Set Element To Zero ==
  u : Inport
  Set Element To Zero : MATLAB Function  TreatAsAtomicUnit=on
  y : Outport  VectorParamsAs1DForOutWhenUnconnected=off
  wires:
  u/1 -> Set Element To Zero/1(u)
  Set Element To Zero/1(y) -> y/1

== system qless_forgetting_factor_16x16_nofifo/MVDR_QLess_HDL/Complex Partial-Systolic Matrix Solve Using Q-less QR Decomposition with Forgetting Factor Manually Tiled n=16/Complex Partial-Systolic Q-less QR with Forgetting Factor/Complex Partial-Systolic Q-less QR with Forgetting Factor Manually tiled/Complex Partial-Systolic Q-less QR Decomposition with Forgetting Factor Section Constant pivot10/Complex Partial-Systolic Q-less QR Row Rotations/Q-less QR Rotate First Element To Real1/Q-less QR Real Row Rotations/Inverse CORDIC Gain ==
  u : Inport
  MATLAB Function : MATLAB Function  TreatAsAtomicUnit=on
  y : Outport  VectorParamsAs1DForOutWhenUnconnected=off
  wires:
  MATLAB Function/1(y) -> y/1
  u/1 -> MATLAB Function/1(u)

== system qless_forgetting_factor_16x16_nofifo/MVDR_QLess_HDL/Complex Partial-Systolic Matrix Solve Using Q-less QR Decomposition with Forgetting Factor Manually Tiled n=16/Complex Partial-Systolic Q-less QR with Forgetting Factor/Complex Partial-Systolic Q-less QR with Forgetting Factor Manually tiled/Complex Partial-Systolic Q-less QR Decomposition with Forgetting Factor Section Constant pivot10/Complex Partial-Systolic Q-less QR Row Rotations/Q-less QR Rotate First Element To Real1/Q-less QR Real Row Rotations/Inverse CORDIC Gain1 ==
  u : Inport
  MATLAB Function : MATLAB Function  TreatAsAtomicUnit=on
  y : Outport  VectorParamsAs1DForOutWhenUnconnected=off
  wires:
  MATLAB Function/1(y) -> y/1
  u/1 -> MATLAB Function/1(u)

== system qless_forgetting_factor_16x16_nofifo/MVDR_QLess_HDL/Complex Partial-Systolic Matrix Solve Using Q-less QR Decomposition with Forgetting Factor Manually Tiled n=16/Complex Partial-Systolic Q-less QR with Forgetting Factor/Complex Partial-Systolic Q-less QR with Forgetting Factor Manually tiled/Complex Partial-Systolic Q-less QR Decomposition with Forgetting Factor Section Constant pivot10/Complex Partial-Systolic Q-less QR Row Rotations/Q-less QR Rotate First Element To Real1/Q-less QR Real Row Rotations/Q-less QR Real Indexed CORDIC Row Rotation ==
  x : Inport
  y : Inport  Port=2
  validIn : Inport  Port=3
  restart : Inport  Port=4
  CORDIC QR Kernel : MATLAB Function  TreatAsAtomicUnit=on
  Delay{1..3,6} (4 alike) : Delay  DelayLength=1
  State Control : StateControl  StateControl=Synchronous
  Unit Delay Enabled Synchronous1 : hdlsllib/Discrete/Unit Delay Enabled Synchronous  InitialCondition=0.0  SampleTime=-1
      settings: SourceProductBaseCode=SL
  Unit Delay Enabled Synchronous4 : hdlsllib/Discrete/Unit Delay Enabled Synchronous  InitialCondition=0.0  SampleTime=-1
      settings: SourceProductBaseCode=SL
  xOut : Outport  VectorParamsAs1DForOutWhenUnconnected=off
  yOut : Outport  Port=2  VectorParamsAs1DForOutWhenUnconnected=off
  validOut : Outport  Port=3  VectorParamsAs1DForOutWhenUnconnected=off
  ready : Outport  Port=4  VectorParamsAs1DForOutWhenUnconnected=off
  wires:
  Delay6/1 -> CORDIC QR Kernel/3(validIn)
  Delay2/1 -> CORDIC QR Kernel/2(yIn)
  Delay1/1 -> CORDIC QR Kernel/1(xIn)
  CORDIC QR Kernel/4(ready) -> ready/1
  CORDIC QR Kernel/3(validOut) -> Unit Delay Enabled Synchronous1/2, Unit Delay Enabled Synchronous4/2, Delay3/1
  restart/1 -> CORDIC QR Kernel/4(restart)
  Unit Delay Enabled Synchronous4/1 -> xOut/1
  validIn/1 -> Delay6/1
  CORDIC QR Kernel/2(yOut) -> Unit Delay Enabled Synchronous1/1
  x/1 -> Delay1/1
  y/1 -> Delay2/1
  CORDIC QR Kernel/1(xOut) -> Unit Delay Enabled Synchronous4/1
  Unit Delay Enabled Synchronous1/1 -> yOut/1
  Delay3/1 -> validOut/1

== system qless_forgetting_factor_16x16_nofifo/MVDR_QLess_HDL/Complex Partial-Systolic Matrix Solve Using Q-less QR Decomposition with Forgetting Factor Manually Tiled n=16/Complex Partial-Systolic Q-less QR with Forgetting Factor/Complex Partial-Systolic Q-less QR with Forgetting Factor Manually tiled/Complex Partial-Systolic Q-less QR Decomposition with Forgetting Factor Section Constant pivot10/Complex Partial-Systolic Q-less QR Row Rotations/Q-less QR Rotate First Element To Real1/Q-less QR Real Row Rotations/Set Element To Zero ==
  u : Inport
  Set Element To Zero : MATLAB Function  TreatAsAtomicUnit=on
  y : Outport  VectorParamsAs1DForOutWhenUnconnected=off
  wires:
  u/1 -> Set Element To Zero/1(u)
  Set Element To Zero/1(y) -> y/1

== system qless_forgetting_factor_16x16_nofifo/MVDR_QLess_HDL/Complex Partial-Systolic Matrix Solve Using Q-less QR Decomposition with Forgetting Factor Manually Tiled n=16/Complex Partial-Systolic Q-less QR with Forgetting Factor/Complex Partial-Systolic Q-less QR with Forgetting Factor Manually tiled/Complex Partial-Systolic Q-less QR Decomposition with Forgetting Factor Section Constant pivot11/Complex Partial-Systolic Q-less QR Row Rotations/Q-less QR Rotate First Element To Real1/Q-less QR Real Row Rotations/Inverse CORDIC Gain ==
  u : Inport
  MATLAB Function : MATLAB Function  TreatAsAtomicUnit=on
  y : Outport  VectorParamsAs1DForOutWhenUnconnected=off
  wires:
  MATLAB Function/1(y) -> y/1
  u/1 -> MATLAB Function/1(u)

== system qless_forgetting_factor_16x16_nofifo/MVDR_QLess_HDL/Complex Partial-Systolic Matrix Solve Using Q-less QR Decomposition with Forgetting Factor Manually Tiled n=16/Complex Partial-Systolic Q-less QR with Forgetting Factor/Complex Partial-Systolic Q-less QR with Forgetting Factor Manually tiled/Complex Partial-Systolic Q-less QR Decomposition with Forgetting Factor Section Constant pivot11/Complex Partial-Systolic Q-less QR Row Rotations/Q-less QR Rotate First Element To Real1/Q-less QR Real Row Rotations/Inverse CORDIC Gain1 ==
  u : Inport
  MATLAB Function : MATLAB Function  TreatAsAtomicUnit=on
  y : Outport  VectorParamsAs1DForOutWhenUnconnected=off
  wires:
  MATLAB Function/1(y) -> y/1
  u/1 -> MATLAB Function/1(u)

== system qless_forgetting_factor_16x16_nofifo/MVDR_QLess_HDL/Complex Partial-Systolic Matrix Solve Using Q-less QR Decomposition with Forgetting Factor Manually Tiled n=16/Complex Partial-Systolic Q-less QR with Forgetting Factor/Complex Partial-Systolic Q-less QR with Forgetting Factor Manually tiled/Complex Partial-Systolic Q-less QR Decomposition with Forgetting Factor Section Constant pivot11/Complex Partial-Systolic Q-less QR Row Rotations/Q-less QR Rotate First Element To Real1/Q-less QR Real Row Rotations/Q-less QR Real Indexed CORDIC Row Rotation ==
  x : Inport
  y : Inport  Port=2
  validIn : Inport  Port=3
  restart : Inport  Port=4
  CORDIC QR Kernel : MATLAB Function  TreatAsAtomicUnit=on
  Delay{1..3,6} (4 alike) : Delay  DelayLength=1
  State Control : StateControl  StateControl=Synchronous
  Unit Delay Enabled Synchronous1 : hdlsllib/Discrete/Unit Delay Enabled Synchronous  InitialCondition=0.0  SampleTime=-1
      settings: SourceProductBaseCode=SL
  Unit Delay Enabled Synchronous4 : hdlsllib/Discrete/Unit Delay Enabled Synchronous  InitialCondition=0.0  SampleTime=-1
      settings: SourceProductBaseCode=SL
  xOut : Outport  VectorParamsAs1DForOutWhenUnconnected=off
  yOut : Outport  Port=2  VectorParamsAs1DForOutWhenUnconnected=off
  validOut : Outport  Port=3  VectorParamsAs1DForOutWhenUnconnected=off
  ready : Outport  Port=4  VectorParamsAs1DForOutWhenUnconnected=off
  wires:
  Delay6/1 -> CORDIC QR Kernel/3(validIn)
  Delay2/1 -> CORDIC QR Kernel/2(yIn)
  Delay1/1 -> CORDIC QR Kernel/1(xIn)
  CORDIC QR Kernel/4(ready) -> ready/1
  CORDIC QR Kernel/3(validOut) -> Unit Delay Enabled Synchronous1/2, Unit Delay Enabled Synchronous4/2, Delay3/1
  restart/1 -> CORDIC QR Kernel/4(restart)
  Unit Delay Enabled Synchronous4/1 -> xOut/1
  validIn/1 -> Delay6/1
  CORDIC QR Kernel/2(yOut) -> Unit Delay Enabled Synchronous1/1
  x/1 -> Delay1/1
  y/1 -> Delay2/1
  CORDIC QR Kernel/1(xOut) -> Unit Delay Enabled Synchronous4/1
  Unit Delay Enabled Synchronous1/1 -> yOut/1
  Delay3/1 -> validOut/1

== system qless_forgetting_factor_16x16_nofifo/MVDR_QLess_HDL/Complex Partial-Systolic Matrix Solve Using Q-less QR Decomposition with Forgetting Factor Manually Tiled n=16/Complex Partial-Systolic Q-less QR with Forgetting Factor/Complex Partial-Systolic Q-less QR with Forgetting Factor Manually tiled/Complex Partial-Systolic Q-less QR Decomposition with Forgetting Factor Section Constant pivot11/Complex Partial-Systolic Q-less QR Row Rotations/Q-less QR Rotate First Element To Real1/Q-less QR Real Row Rotations/Set Element To Zero ==
  u : Inport
  Set Element To Zero : MATLAB Function  TreatAsAtomicUnit=on
  y : Outport  VectorParamsAs1DForOutWhenUnconnected=off
  wires:
  u/1 -> Set Element To Zero/1(u)
  Set Element To Zero/1(y) -> y/1

== system qless_forgetting_factor_16x16_nofifo/MVDR_QLess_HDL/Complex Partial-Systolic Matrix Solve Using Q-less QR Decomposition with Forgetting Factor Manually Tiled n=16/Complex Partial-Systolic Q-less QR with Forgetting Factor/Complex Partial-Systolic Q-less QR with Forgetting Factor Manually tiled/Complex Partial-Systolic Q-less QR Decomposition with Forgetting Factor Section Constant pivot12/Complex Partial-Systolic Q-less QR Row Rotations/Q-less QR Rotate First Element To Real1/Q-less QR Real Row Rotations/Inverse CORDIC Gain ==
  u : Inport
  MATLAB Function : MATLAB Function  TreatAsAtomicUnit=on
  y : Outport  VectorParamsAs1DForOutWhenUnconnected=off
  wires:
  MATLAB Function/1(y) -> y/1
  u/1 -> MATLAB Function/1(u)

== system qless_forgetting_factor_16x16_nofifo/MVDR_QLess_HDL/Complex Partial-Systolic Matrix Solve Using Q-less QR Decomposition with Forgetting Factor Manually Tiled n=16/Complex Partial-Systolic Q-less QR with Forgetting Factor/Complex Partial-Systolic Q-less QR with Forgetting Factor Manually tiled/Complex Partial-Systolic Q-less QR Decomposition with Forgetting Factor Section Constant pivot12/Complex Partial-Systolic Q-less QR Row Rotations/Q-less QR Rotate First Element To Real1/Q-less QR Real Row Rotations/Inverse CORDIC Gain1 ==
  u : Inport
  MATLAB Function : MATLAB Function  TreatAsAtomicUnit=on
  y : Outport  VectorParamsAs1DForOutWhenUnconnected=off
  wires:
  MATLAB Function/1(y) -> y/1
  u/1 -> MATLAB Function/1(u)
